simulink model "moment_ul"  (R2018b)
settings: Solver=VariableStepAuto  StartTime=0.0  StopTime=10.0  RelTol=1e-3
libraries: vrlib x1
settings Model: Creator=mcobb  LastModifiedBy=mcobb

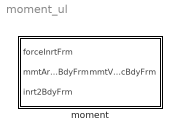
== system moment_ul ==
  moment : Subsystem

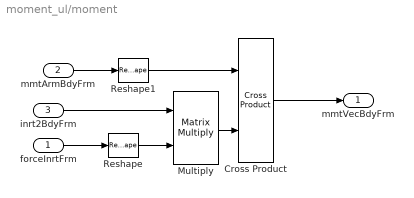
== system moment_ul/moment ==
  forceInrtFrm : Inport
  mmtArmBdyFrm : Inport  Port=2
  inrt2BdyFrm : Inport  Port=3
  Cross Product : vrlib/Utilities/Cross Product
      settings: SourceProductBaseCode=VR
  Multiply : Product  Multiplication=Matrix(*)
  Reshape : Reshape  OutputDimensionality=Column vector (2-D)
  Reshape1 : Reshape  OutputDimensionality=Column vector (2-D)
  mmtVecBdyFrm : Outport
  wires:
  forceInrtFrm/1 -> Reshape/1
  inrt2BdyFrm/1 -> Multiply/1
  Multiply/1 -> Cross Product/2
  mmtArmBdyFrm/1 -> Reshape1/1
  Cross Product/1 -> mmtVecBdyFrm/1
  Reshape/1 -> Multiply/2
  Reshape1/1 -> Cross Product/1
